simulink model "Prac_2_Q1_1"  (R2021a)
settings: Solver=FixedStepAuto  StartTime=0.0  StopTime=7  FixedStep=0.02  RelTol=1e-3
values from neighbouring files (symbols this model uses):
  inputAmp = 50    [Prac_2.m]
  inputBias = 40    [Prac_2.m]
  rangeMax = 115    [Prac_2.m]
  rangeMin = -15    [Prac_2.m]
  sampleTime = 0.02    [Prac_2.m]
  Sens = 45.9/1000    (= 0.0459)    [Prac_2.m]
libraries: simulink x1, simulink_extras x1, cstblocks x1
settings Model: Creator=kaibr  LastModifiedBy=mluser
settings SolverCC: AlgebraicLoopSolver=TrustRegion
settings DebuggingCC: SFMachineParentedDataDiag=warning

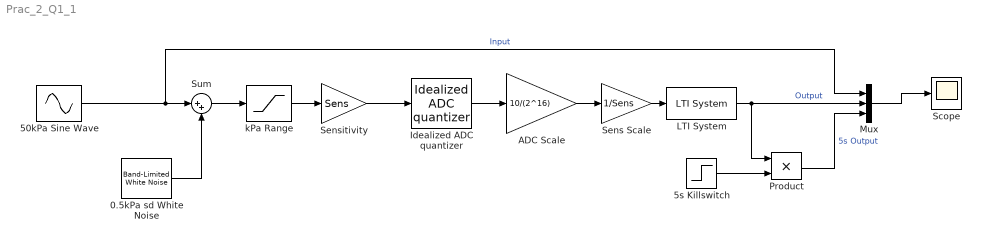
== system Prac_2_Q1_1 ==
  0.5kPa sd White Noise : simulink/Sources/Band-Limited White Noise  Cov=noisePow  Ts=sampleTime  seed=[23341]
  50kPa Sine Wave : Sin  Amplitude=inputAmp  Bias=inputBias  Frequency=0.5  SampleTime=sampleTime
  5s Killswitch : Step  Time=5  Before=1  After=0  SampleTime=sampleTime
  ADC Scale : Gain  Gain=10/(2^16)
  Idealized ADC quantizer : simulink_extras/Additional Discrete/Idealized ADC quantizer  NumberOfConverterBits=16  Vmin=-5  Vmax=5  OutputDataType=double  OutputNegativeValues=on
  LTI System : cstblocks/LTI System  sys=delayFn2  IC=[]
  Mux : Mux  Inputs=3
  Product : Product
  Scope : Scope
  Sens Scale : Gain  Gain=1/Sens
  Sensitivity : Gain  Gain=Sens
  Sum : Sum  Inputs=|++
  kPa Range : Saturate  UpperLimit=rangeMax  LowerLimit=rangeMin
  wires:
  Mux/1 -> Scope/1
  0.5kPa sd White Noise/1 -> Sum/2
  Sum/1 -> kPa Range/1
  kPa Range/1 -> Sensitivity/1
  Idealized ADC quantizer/1 -> ADC Scale/1
  Sens Scale/1 -> LTI System/1
  ADC Scale/1 -> Sens Scale/1
  Sensitivity/1 -> Idealized ADC quantizer/1
  50kPa Sine Wave/1 -> Mux/1, Sum/1  "Input"
  LTI System/1 -> Mux/2, Product/1  "Output"
  5s Killswitch/1 -> Product/2
  Product/1 -> Mux/3  "5s Output"
